simulink model "IRlineFollowInitialVersion1"  (R2023b)
settings: Solver=FixedStepAuto  StartTime=0.0  StopTime=inf  RelTol=1e-3  EnableMultiTasking=on
libraries: vexarmcortexlib x5
settings Model: Creator=ierdn  LastModifiedBy=ierdn
settings DataIOCC: LimitDataPoints=on  SignalLoggingSaveFormat=ModelDataLogs  ReturnWorkspaceOutputs=off
settings OptimizationCC: ExpressionDepthLimit=2147483647  LifeSpan=Inf  MaxStackSize=64  EfficientTunableParamExpr=on
settings DebuggingCC: UnderspecifiedInitializationDetection=Classic  MergeDetectMultiDrivingBlocksExec=none  InheritedTsInSrcMsg=none  FcnCallInpInsideContextMsg=warning  StateNameClashWarn=warning  SFUnexpectedBacktrackingDiag=warning  SFNoUnconditionalDefaultTransitionDiag=warning  SFExecutionAtInitializationDiag=none  ArithmeticOperatorsInVariantConditions=warning
settings HardwareCC: ProdBitPerPointer=32  ProdBitPerSizeT=32  ProdBitPerPtrDiffT=32  ProdLargestAtomicInteger=Long  ProdLargestAtomicFloat=Double  ProdIntDivRoundTo=Undefined  ProdWordSize=32  ProdHWDeviceType=ARM Compatible->ARM Cortex
settings ModelReferenceCC: EnableRefExpFcnMdlSchedulingChecks=on  PropagateSignalLabelsOutOfModel=off
settings SFSimCC: MATLABDynamicMemAlloc=off  CustomCodeUndefinedFunction=UseInterfaceOnly
settings RTWCC: Description=Embedded Coder  SystemTargetFile=ert.tlc  HardwareBoard=ARM Cortex-based VEX Microcontroller  TemplateMakefile=ert_default_tmf  Toolchain=GNU Tools for VEX ARM Cortex
settings CodeAppCC: IgnoreCustomStorageClasses=off  CustomSymbolStrType=$N$R$M  StateflowObjectComments=on  InternalIdentifier=Classic
settings ERTTargetCC: CodeReplacementLibrary=GCC ARM Cortex-M3  MultiwordLength=2048  ConvertIfToSwitch=off  SuppressUnreachableDefaultCases=off

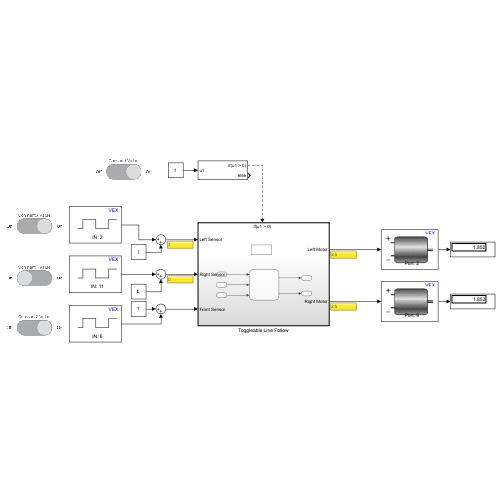
[thumbnail: Simulink's stored preview of the top-level diagram]
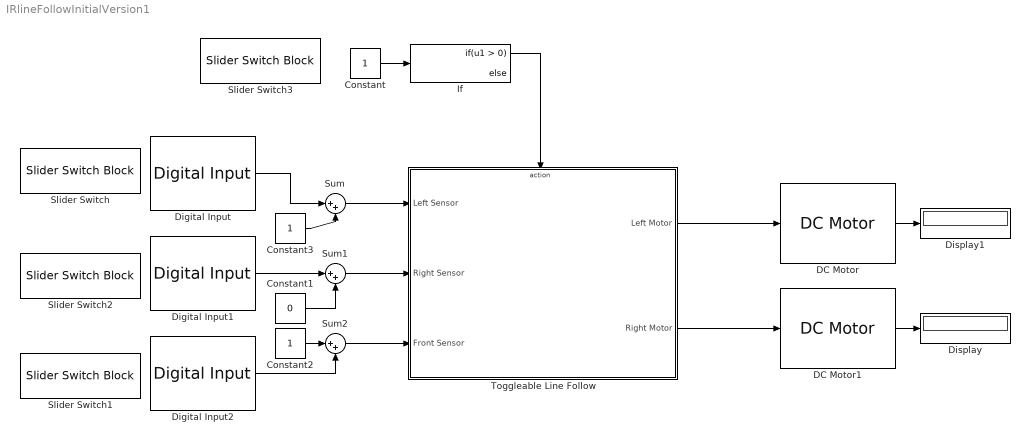
== system IRlineFollowInitialVersion1 ==
  Constant : Constant
  Constant1 : Constant  Value=0
  Constant2 : Constant
  Constant3 : Constant
  DC Motor : vexarmcortexlib/Actuators/DC Motor  motor=2  scaleFactor=1/13.5  SimulationOut=on
  DC Motor1 : vexarmcortexlib/Actuators/DC Motor  motor=9  scaleFactor=1/13.5  SimulationOut=on
  Digital Input : vexarmcortexlib/Sensors/Digital Input  inChan=2  SimulationIn=off  SampleTime=0.2
  Digital Input1 : vexarmcortexlib/Sensors/Digital Input  inChan=11  SimulationIn=off  SampleTime=0.2
  Digital Input2 : vexarmcortexlib/Sensors/Digital Input  inChan=6  SimulationIn=off  SampleTime=0.2
  Display : Display
  Display1 : Display
  If : If
  Slider Switch{,1..3} (4 alike) : SliderSwitchBlock
      settings: Values={{'Off', 'On'}, [0 1]}
  Sum : Sum  Inputs=|++
  Sum1 : Sum  Inputs=|++
  Sum2 : Sum  Inputs=|++
  Toggleable Line Follow : Subsystem  TreatAsAtomicUnit=on
  wires:
  Constant/1 -> If/1
  If/1 -> Toggleable Line Follow/Action
  Digital Input1/1 -> Sum1/1
  Toggleable Line Follow/1(Left Motor) -> DC Motor/1
  Toggleable Line Follow/2(Right Motor) -> DC Motor1/1
  DC Motor1/1 -> Display/1
  DC Motor/1 -> Display1/1
  Constant3/1 -> Sum/2
  Digital Input/1 -> Sum/1
  Sum/1 -> Toggleable Line Follow/1(Left Sensor)
  Constant1/1 -> Sum1/2
  Sum1/1 -> Toggleable Line Follow/2(Right Sensor)
  Digital Input2/1 -> Sum2/2
  Sum2/1 -> Toggleable Line Follow/3(Front Sensor)
  Constant2/1 -> Sum2/1

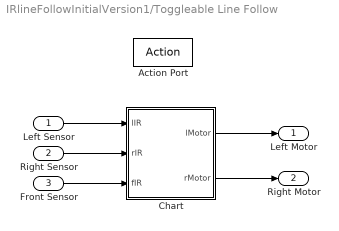
== system IRlineFollowInitialVersion1/Toggleable Line Follow ==
  Left Sensor : Inport
  Right Sensor : Inport  Port=2
  Front Sensor : Inport  Port=3
  Action Port : ActionPort  ActionPortLabel=if(u1 > 0)
  Chart : Stateflow chart  TreatAsAtomicUnit=on
      settings: PortSchema="{\"entries\":[{\"content\":{\"sides\":[{\"content\":{\"connectorIds\":[\"In2\",\"In3\",\"In1\"]},\"type\":\"ConnectorPlacement.EquallySpacedRectSide\",\"uuid\":\"247074c7-d082-4199-9f42-5ee7f9b2f2c5\"},{\"content\":{\"connectorIds\":[\"Out1\",\"Out2\"],\"side\":\"RIGHT\"},\"type\":\"ConnectorPlacement.EquallySpacedRectSide\",\"uuid\":\"36e2493d-b1f5-4e64-901d-97da90bd168d\"},{\"content\":{\"side\":\"TOP\"},\"type\":\"ConnectorPlacement.EquallySpacedRectSide\",\"uuid\":\"46c427ed-bb7b-4aa4-a673-b474e6d6a53a\"}]},\"type\":\"ConnectorPlacement.EquallySpacedConnector\",\"uuid\":\"23614380-3184-4867-9eb4-661b2749fd08\"}],\"packageUris\":[\"http://schema.mathworks.com/mf0/Connector/R2020b\"],\"version\":\"1.0\"}"
  Left Motor : Outport
  Right Motor : Outport  Port=2
  wires:
  Left Sensor/1 -> Chart/2(lIR)
  Front Sensor/1 -> Chart/1(fIR)
  Right Sensor/1 -> Chart/3(rIR)
  Chart/1(lMotor) -> Left Motor/1
  Chart/2(rMotor) -> Right Motor/1

== stateflow chart IRlineFollowInitialVersion1/Toggleable Line Follow/Chart ==
  state Follow
    Forward;
  state Middle
    lMotor = 0;
    rMotor = 0;
  state Start
    brainDetect = 0;
    slow = 1;
  Middle -> Follow : [brainDetect == 0]
  (default) -> Start
  Start -> Middle
  Follow -> Middle : [after(1,sec)&&brainDetect == 1]
  data: fIR input; lIR input; rIR input; lMotor output [-127..127] =50; rMotor output [-127..127] =50; brainDetect local [0..1] =0; slow local
  function Forward:
    | function Forward
    | 
    | init();
    | 
    | lIREQ0 = false;
    | rIREQ0 = false;
    | fIREQ0 = false;
    | 
    | 
    | % Left IR is equal to 0 should be 1
    | 
    | lIREQ0 = logical(lIR == 0);
    | 
    | % Right IR is equal to 0 should be 0
    | 
    | rIREQ0 = logical(rIR == 0);
    | 
    | % Front IR is equal to 0
    | 
    | fIREQ0 = logical(fIR == 0);
    | 
    | if (~lIREQ0 && rIREQ0 && ~fIREQ0)
    |     A5();
    | elseif (lIREQ0 && ~rIREQ0 && ~fIREQ0)
    |     A2();
    | elseif (lIREQ0 && rIREQ0 && ~fIREQ0)
    |     A2();
    | elseif (~lIREQ0 && ~rIREQ0 && ~fIREQ0)
    |     A3();
    | elseif (~lIREQ0 && ~rIREQ0 && fIREQ0)
    |     A4();
    | elseif (lIREQ0 && ~rIREQ0 && fIREQ0)
    |     A4();
    | elseif (lIREQ0 && rIREQ0 && fIREQ0)
    |     A4();
    | else % Default
    |     A4();
    | end
    | 
    | function init()
    | 
    | % Initial Speed
    | 
    | lMotor = 50/slow;
    | rMotor = 50/slow;
    | 
    | function A2()
    | 
    | % Left IR is seeing white - turn Left
    | 
    | lMotor = 25/slow;
    | 
    | function A3()
    | 
    | % Right IR is seeing black - turn Right
    | 
    | rMotor = 25/slow;
    | 
    | function A4()
    | 
    | % fIR is seeing the brain and the sensors are alighned - Stop
    | 
    | rMotor = 0;
    | lMotor = 0;
    | brainDetect = 1;
    | 
    | function A5()
    | 
    | % Everything is good
    | 
    | rMotor = 50/slow;
    | rMotor = 50/slow;
